simulink model "narx"  (R2019a)
settings: Solver=VariableStepAuto  StartTime=0.0  StopTime=10.0  RelTol=1e-3
libraries: neural x208
(part 3 of 4)

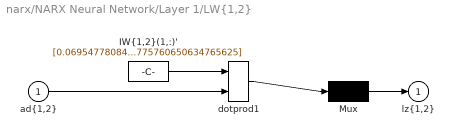
== system narx/NARX Neural Network/Layer 1/LW{1,2} ==
  "ad{1,2}" : Inport  PortDimensions=400  SampleTime=0.1
      mask Display: e = 0.06;c1 = [120 230 180]/255;c2 = ([120 230 180]+0)/(256+128);c3 = ([120 230 180]+128)/(256+128);patch([0 1 1 0],[0 0 1 1],c1);patch([0 1 1 1-e 1-e 0+e],[0 0 1 1-e 0+e 0+e],c2);patch([0 0 1 1-e 0+e 0+e],[0 1 1 1-e 1-e 0+e],c3);plot([0 1 1 0 0],[0 0 1 1 0]);
  "IW{1,2}(1,:)'" : Constant  Value=[0.06954778084371961155429886503043235279619693756103515625;-0.043032984621073612496733318266706191934645175933837890625;-0.0877202419060049976007320537974010221660137176513671875;0.03711809287507895904756338723018416203558444976806640625;0.05131876970590155961904343939750106073915958404541015625;-0.0238131694780161114188832272020590608008205890655517578125;-0.033690668054631507655205524542907369323074817657470703125;0.06581807560963852388180583830035175196826457977294921875;-0.00801812581178163417960913506021825014613568782806396484375;0.070802936021443108050021919552818872034549713134765625;0.027480357214325255854614482586839585565030574798583984375;-0.06751110573486705790369200030909269116818904876708984375;-0.01010291500685255895730652042630026699043810367584228515625;-0.030651203953214599395860062713836668990552425384521484375;0.050502583361956947249904459340541507117450237274169921875;0.00213145965090496582183821061562412069179117679595947265625;-0.07220686877646766144156487143845879472792148590087890625;-0.0102924462220746644469659969445274327881634235382080078125;0.07770445080335268428495254511290113441646099090576171875;-0.01155690922746742919924312076318528852425515651702880859375;-0.06162141318948714807657296432807925157248973846435546875;0.01202643992945601723876247746147782891057431697845458984375;0.07644541092298705320384755168561241589486598968505859375;0.057818243945609693046350230360985733568668365478515625;-0.07417710177828153172985281571527593769133090972900390625;0.059591486666174586783739641759893856942653656005859375;0.07438413178966618577447889038012363016605377197265625;0.0828152743328926244092969000121229328215122222900390625;0.051460094830914480945605049555524601601064205169677734375;-0.046124889637994714863822309780516661703586578369140625;-0.0429422579564297801635319729030015878379344940185546875;-0.07083938829556445104795869838198996149003505706787109375;-0.03889465285627792534572932936498546041548252105712890625;-0.06115377227675948546004036643353174440562725067138671875;0.038302200933641283864261595226707868278026580810546875;-0.0123448681274885112280070842416535015217959880828857421875;0.039488343689792350377221197277322062291204929351806640625;0.08417867561418156119312783403074718080461025238037109375;0.053916683617023099250875617372003034688532352447509765625;0.0109248704105002793218748280423824326135218143463134765625;-0.0036864689960412785722787543107870078529231250286102294921875;-0.048604416570240026318483472778098075650632381439208984375;-0.062473038777278777633483741738018579781055450439453125;0.035434571202584759508358303037311998195946216583251953125;0.01503603219799232691700208164320429204963147640228271484375;4.80253056802357574371110937594409051598631776869297027587890625e-05;0.056839158486344111553822955329451360739767551422119140625;-0.0399331012067128676701344147659256123006343841552734375;-0.0022393530646860073350656872293029664433561265468597412109375;-0.07060200930107141115144031573436222970485687255859375;-0.032258384380879190356239405446103774011135101318359375;0.0247762759830111624348436549780672066844999790191650390625;0.06294795172204160904616543348311097361147403717041015625;0.043056609638628083602807095076059340499341487884521484375;0.051686529063135068506884550743052386678755283355712890625;-0.00616880889515120968413786073369919904507696628570556640625;-0.039732113460623684486616724598206928931176662445068359375;-0.01048147127721324282922932269457305665127933025360107421875;-0.03929683273630869833059620077619911171495914459228515625;-0.02714702938880438065627487276287865824997425079345703125;0.01721241226468329943433133166763582266867160797119140625;-0.0172343463322831881578967028190163546241819858551025390625;0.07068491720488878637951302152941934764385223388671875;-0.0334444569918347645032241644003079272806644439697265625;0.041132666153089296467992852512907120399177074432373046875;-0.053510862624672229925781863357769907452166080474853515625 ...(+19948 chars)]
      mask Display: e = 0.06;c1 = [120 150 230]/255;c2 = ([120 150 230]+0)/383;c3 = ([120 150 230]+128)/383;patch([0 1 1 0],[0 0 1 1],c1);patch([0 1 1 1-e 1-e 0+e],[0 0 1 1-e 0+e 0+e],c2);patch([0 0 1 1-e 0+e 0+e],[0 1 1 1-e 1-e 0+e],c3);plot([0 1 1 0 0],[0 0 1 1 0]);disp('weights');
  Mux : Mux  Inputs=1
      mask Display: e = 0.06;c1 = [120 150 230]/255;c2 = ([120 150 230]+0)/383;c3 = ([120 150 230]+128)/383;patch([0 1 1 0],[0 0 1 1],c1);patch([0 1 1 1-e 1-e 0+e],[0 0 1 1-e 0+e 0+e],c2);patch([0 0 1 1-e 0+e 0+e],[0 1 1 1-e 1-e 0+e],c3);plot([0 1 1 0 0],[0 0 1 1 0]);disp('Mux');
  dotprod1 : neural/Weight Functions/dotprod
      settings: SourceProductName=MATLAB Runtime - Deep Learning Toolbox  SourceProductBaseCode=Missing
  "lz{1,2}" : Outport
      mask Display: e = 0.06;c1 = [120 230 180]/255;c2 = ([120 230 180]+0)/(256+128);c3 = ([120 230 180]+128)/(256+128);patch([0 1 1 0],[0 0 1 1],c1);patch([0 1 1 1-e 1-e 0+e],[0 0 1 1-e 0+e 0+e],c2);patch([0 0 1 1-e 0+e 0+e],[0 1 1 1-e 1-e 0+e],c3);plot([0 1 1 0 0],[0 0 1 1 0]);
  wires:
  "IW{1,2}(1,:)'"/1 -> dotprod1/1
  "ad{1,2}"/1 -> dotprod1/2
  dotprod1/1 -> Mux/1
  Mux/1 -> "lz{1,2}"/1

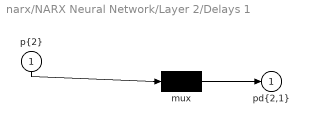
== system narx/NARX Neural Network/Layer 2/Delays 1 ==
  "p{2}" : Inport  PortDimensions=1  SampleTime=0.1
      mask Display: e = 0.06;c1 = [120 230 180]/255;c2 = ([120 230 180]+0)/(256+128);c3 = ([120 230 180]+128)/(256+128);patch([0 1 1 0],[0 0 1 1],c1);patch([0 1 1 1-e 1-e 0+e],[0 0 1 1-e 0+e 0+e],c2);patch([0 0 1 1-e 0+e 0+e],[0 1 1 1-e 1-e 0+e],c3);plot([0 1 1 0 0],[0 0 1 1 0]);
  mux : Mux  Inputs=1
      mask Display: e = 0.06;c1 = [120 150 230]/255;c2 = ([120 150 230]+0)/383;c3 = ([120 150 230]+128)/383;patch([0 1 1 0],[0 0 1 1],c1);patch([0 1 1 1-e 1-e 0+e],[0 0 1 1-e 0+e 0+e],c2);patch([0 0 1 1-e 0+e 0+e],[0 1 1 1-e 1-e 0+e],c3);plot([0 1 1 0 0],[0 0 1 1 0]);disp('Mux')
  "pd{2,1}" : Outport
      mask Display: e = 0.06;c1 = [120 230 180]/255;c2 = ([120 230 180]+0)/(256+128);c3 = ([120 230 180]+128)/(256+128);patch([0 1 1 0],[0 0 1 1],c1);patch([0 1 1 1-e 1-e 0+e],[0 0 1 1-e 0+e 0+e],c2);patch([0 0 1 1-e 0+e 0+e],[0 1 1 1-e 1-e 0+e],c3);plot([0 1 1 0 0],[0 0 1 1 0]);
  wires:
  "p{2}"/1 -> mux/1
  mux/1 -> "pd{2,1}"/1
